simulink model "Robot_model_PD_control"  (Simulink 7.8)
settings: Solver=ode1  StartTime=0.0  StopTime=1  FixedStep=.001  RelTol=1e-3
undefined symbols (not defined in the file or in its folder): inert, Xdsim
settings Model: Creator=Administrator  LastModifiedBy=Christian Hoffmann
settings DataIOCC: LimitDataPoints=off  SaveOutput=off  SaveTime=off
settings OptimizationCC: InitFltsAndDblsToZero=on
settings DebuggingCC: SaveWithParameterizedLinksMsg=none  SignalResolutionControl=TryResolveAllWithWarning  SolverPrmCheckMsg=none  MultiTaskDSMMsg=warning  MultiTaskCondExecSysMsg=none  FcnCallInpInsideContextMsg=Use local settings  StrictBusMsg=Warning
settings HardwareCC: TargetUnknown=on
settings SFSimCC: SimParseCustomCode=off
settings RTWCC: IncludeERTFirstTime=on
settings GRTTargetCC: TargetFcnLib=ansi_tfl_tmw.mat

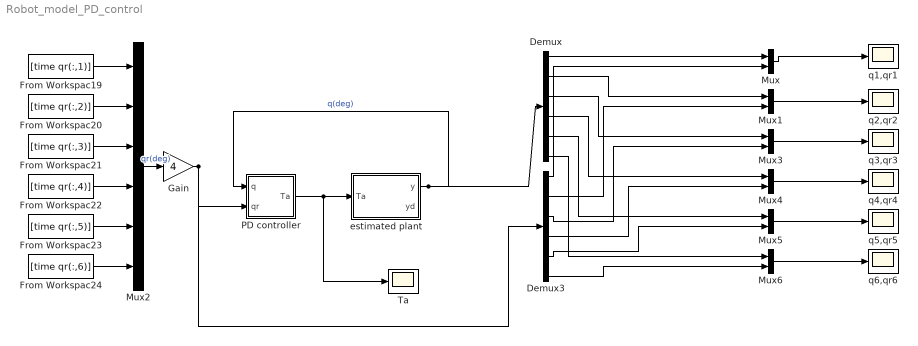
== system Robot_model_PD_control ==
  Demux : Demux  Outputs=6
  Demux3 : Demux  Outputs=6
  From Workspac19 : FromWorkspace  VariableName=[time qr(:,1)]  SampleTime=0
  From Workspac20 : FromWorkspace  VariableName=[time qr(:,2)]  SampleTime=0
  From Workspac21 : FromWorkspace  VariableName=[time qr(:,3)]  SampleTime=0
  From Workspac22 : FromWorkspace  VariableName=[time qr(:,4)]  SampleTime=0
  From Workspac23 : FromWorkspace  VariableName=[time qr(:,5)]  SampleTime=0
  From Workspac24 : FromWorkspace  VariableName=[time qr(:,6)]  SampleTime=0
  Gain : Gain  Gain=4
  Mux{,1,3..6} (6 alike) : Mux  Inputs=2
  Mux2 : Mux  Inputs=6
  PD controller : Subsystem
  Ta : Scope
      settings: YMin=-50  YMax=225  SaveName=ScopeData6
  estimated plant : Subsystem
  q1,qr1 : Scope
      settings: YMin=-14  YMax=0
  q2,qr2 : Scope
      settings: YMin=-75  YMax=-10  SaveName=q2qr2
  q3,qr3 : Scope
      settings: TimeRange=3  YMin=-0.025  YMax=0.375  SaveName=q3qr3
  q4,qr4 : Scope
      settings: YMin=29  YMax=43  SaveName=ScopeData3
  q5,qr5 : Scope
      settings: YMin=-50  YMax=50  SaveName=ScopeData4
  q6,qr6 : Scope
      settings: YMin=-60  YMax=45  SaveName=ScopeData5
  wires:
  Mux2/1 -> Gain/1  "qr(deg)"
  estimated plant/1(y) -> PD controller/1(q), Demux/1  "q(deg)"
  Demux/1 -> Mux/1
  Demux/2 -> Mux1/1
  Demux/3 -> Mux3/1
  Demux/4 -> Mux4/1
  Demux/5 -> Mux5/1
  Demux/6 -> Mux6/1
  Demux3/6 -> Mux6/2
  Demux3/5 -> Mux5/2
  Demux3/4 -> Mux4/2
  Demux3/3 -> Mux3/2
  Demux3/2 -> Mux1/2
  Demux3/1 -> Mux/2
  Mux/1 -> q1,qr1/1
  Mux1/1 -> q2,qr2/1
  Mux3/1 -> q3,qr3/1
  Mux4/1 -> q4,qr4/1
  Mux5/1 -> q5,qr5/1
  Mux6/1 -> q6,qr6/1
  PD controller/1(Ta) -> estimated plant/1(Ta), Ta/1
  From Workspac19/1 -> Mux2/1
  From Workspac20/1 -> Mux2/2
  From Workspac21/1 -> Mux2/3
  From Workspac22/1 -> Mux2/4
  From Workspac23/1 -> Mux2/5
  From Workspac24/1 -> Mux2/6
  Gain/1 -> PD controller/2(qr), Demux3/1

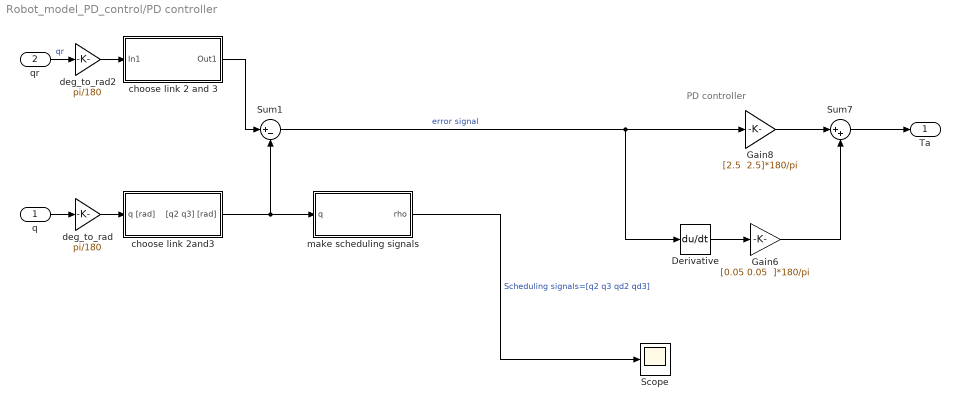
== system Robot_model_PD_control/PD controller ==
  note: PD controller
  q : Inport
  qr : Inport  Port=2
  Derivative : Derivative
  Gain6 : Gain  Gain="[0.05 0.05  ]*180/pi"
      settings: AttributesFormatString=D gain
  Gain8 : Gain  Gain="[2.5  2.5]*180/pi"
      settings: AttributesFormatString=P gain
  Scope : Scope
      settings: SaveName=ScopeData7
  Sum1 : Sum  Inputs=|+-
  Sum7 : Sum  Inputs=|++
  choose link 2 and 3 : Subsystem
  choose link 2and3 : Subsystem
  deg_to_rad : Gain  Gain=pi/180
  deg_to_rad2 : Gain  Gain=pi/180
  make scheduling signals : Subsystem
  Ta : Outport
  wires:
  Gain8/1 -> Sum7/1
  Derivative/1 -> Gain6/1
  Gain6/1 -> Sum7/2
  q/1 -> deg_to_rad/1
  Sum1/1 -> Derivative/1, Gain8/1  "error signal"
  Sum7/1 -> Ta/1
  qr/1 -> deg_to_rad2/1  "qr"
  make scheduling signals/1(rho) -> Scope/1  "Scheduling signals=[q2 q3 qd2 qd3]"
  choose link 2 and 3/1(Out1) -> Sum1/1
  choose link 2and3/1("[q2 q3] [rad]") -> Sum1/2, make scheduling signals/1(q)
  deg_to_rad/1 -> choose link 2and3/1(q [rad])
  deg_to_rad2/1 -> choose link 2 and 3/1(In1)

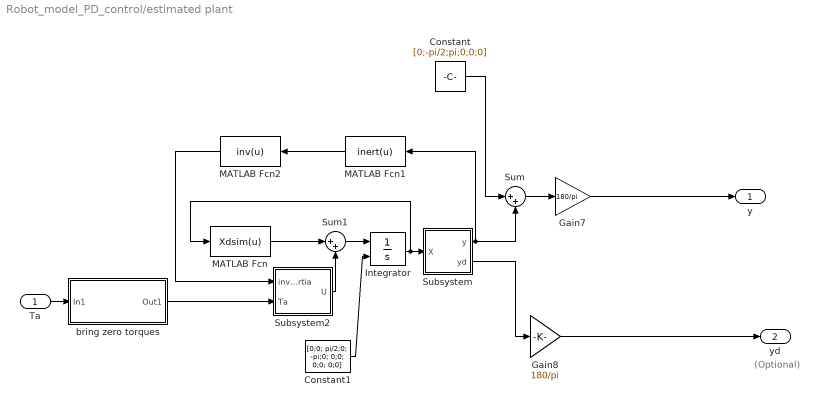
== system Robot_model_PD_control/estimated plant ==
  note: (Optional)
  Ta : Inport
  Constant : Constant  Value=[0;-pi/2;pi;0;0;0]
  Constant1 : Constant  Value="[0;0;    pi/2;0;    -pi;0;    0;0;    0;0;    0;0]"
      settings: AttributesFormatString=initial states, ready position
  Gain7 : Gain  Gain=180/pi
  Gain8 : Gain  Gain=180/pi
  Integrator : Integrator  InitialConditionSource=external
  MATLAB Fcn : MATLABFcn  MATLABFcn=Xdsim(u)
  MATLAB Fcn1 : MATLABFcn  MATLABFcn=inert(u)  Output1D=off
  MATLAB Fcn2 : MATLABFcn  MATLABFcn=inv(u)  Output1D=off
  Subsystem : Subsystem
  Subsystem2 : Subsystem
  Sum : Sum  Inputs=|++
  Sum1 : Sum  Inputs=|++
  bring zero torques : Subsystem
  y : Outport
  yd : Outport  Port=2
  wires:
  Sum/1 -> Gain7/1
  Constant/1 -> Sum/1
  Constant1/1 -> Integrator/2
  Integrator/1 -> MATLAB Fcn/1, Subsystem/1(X)
  Subsystem/2(yd) -> Gain8/1
  Subsystem/1(y) -> MATLAB Fcn1/1, Sum/2
  Sum1/1 -> Integrator/1
  MATLAB Fcn/1 -> Sum1/1
  Subsystem2/1("U ") -> Sum1/2
  MATLAB Fcn2/1 -> Subsystem2/1(inv inertia)
  Gain8/1 -> yd/1
  Gain7/1 -> y/1
  MATLAB Fcn1/1 -> MATLAB Fcn2/1
  Ta/1 -> bring zero torques/1(In1)
  bring zero torques/1(Out1) -> Subsystem2/2(Ta)

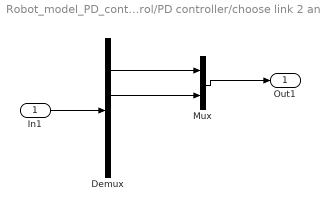
== system Robot_model_PD_control/PD controller/choose link 2 and 3 ==
  In1 : Inport
  Demux : Demux  Outputs=6
  Mux : Mux  Inputs=2
  Out1 : Outport
  wires:
  In1/1 -> Demux/1
  Mux/1 -> Out1/1
  Demux/3 -> Mux/2
  Demux/2 -> Mux/1

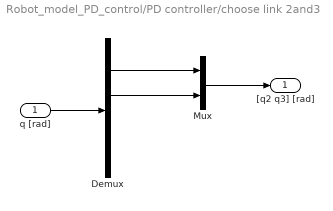
== system Robot_model_PD_control/PD controller/choose link 2and3 ==
  q [rad] : Inport
  Demux : Demux  Outputs=6
  Mux : Mux  Inputs=2
  "[q2 q3] [rad]" : Outport
  wires:
  Demux/2 -> Mux/1
  Demux/3 -> Mux/2
  Mux/1 -> "[q2 q3] [rad]"/1
  q [rad]/1 -> Demux/1

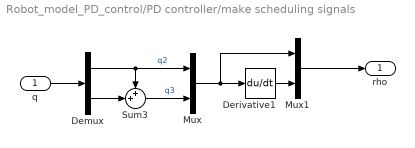
== system Robot_model_PD_control/PD controller/make scheduling signals ==
  q : Inport
  Demux : Demux  Outputs=2
  Derivative1 : Derivative
  Mux : Mux  Inputs=2
  Mux1 : Mux  Inputs=2
  Sum3 : Sum  Inputs=++|
  rho : Outport
  wires:
  Demux/1 -> Mux/1, Sum3/1  "q2"
  Sum3/1 -> Mux/2  "q3"
  Demux/2 -> Sum3/2
  Mux/1 -> Derivative1/1, Mux1/1
  Derivative1/1 -> Mux1/2
  Mux1/1 -> rho/1
  q/1 -> Demux/1

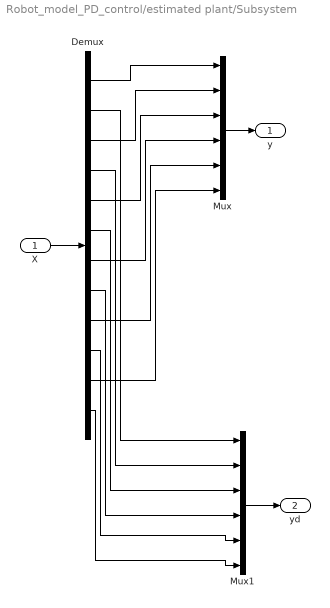
== system Robot_model_PD_control/estimated plant/Subsystem ==
  X : Inport
  Demux : Demux  Outputs=12
  Mux : Mux  Inputs=6
  Mux1 : Mux  Inputs=6
  y : Outport
  yd : Outport  Port=2
  wires:
  Demux/2 -> Mux1/1
  Demux/4 -> Mux1/2
  Demux/6 -> Mux1/3
  Demux/8 -> Mux1/4
  Demux/10 -> Mux1/5
  Demux/12 -> Mux1/6
  Demux/11 -> Mux/6
  Demux/9 -> Mux/5
  Demux/7 -> Mux/4
  Demux/5 -> Mux/3
  Demux/3 -> Mux/2
  Demux/1 -> Mux/1
  Mux/1 -> y/1
  Mux1/1 -> yd/1
  X/1 -> Demux/1

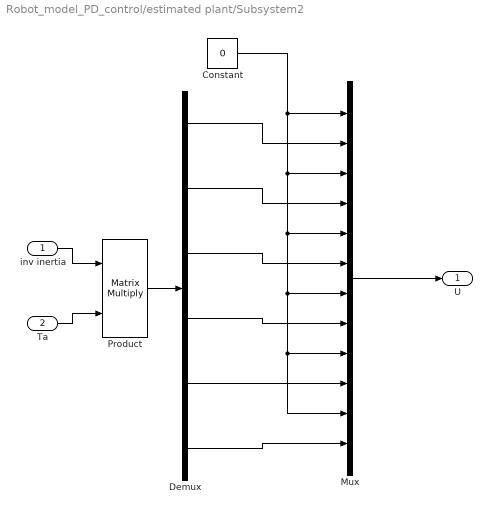
== system Robot_model_PD_control/estimated plant/Subsystem2 ==
  inv inertia : Inport
  Ta : Inport  Port=2
  Constant : Constant  Value=0
  Demux : Demux  Outputs=6
  Mux : Mux  Inputs=12
  Product : Product  Multiplication=Matrix(*)  RndMeth=Zero
  "U " : Outport
  wires:
  Constant/1 -> Mux/11, Mux/9, Mux/7, Mux/5, Mux/3, Mux/1
  Demux/6 -> Mux/12
  Demux/5 -> Mux/10
  Demux/4 -> Mux/8
  Demux/3 -> Mux/6
  Demux/2 -> Mux/4
  Demux/1 -> Mux/2
  Product/1 -> Demux/1
  Ta/1 -> Product/2
  inv inertia/1 -> Product/1
  Mux/1 -> "U "/1

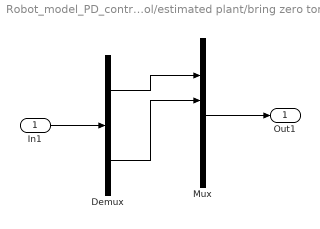
== system Robot_model_PD_control/estimated plant/bring zero torques ==
  In1 : Inport
  Demux : Demux  Outputs=2
  Mux : Mux  Inputs=6
  Out1 : Outport
  wires:
  In1/1 -> Demux/1
  Mux/1 -> Out1/1
  Demux/1 -> Mux/2
  Demux/2 -> Mux/3
